simulink model "ChristmasLights"  (R2021a)
settings: Solver=FixedStepDiscrete  StartTime=0.0  StopTime=40.0  FixedStep=0.050  RelTol=1e-3
settings Model: EnablePacing=on  Creator=ncleju  LastModifiedBy=ncleju

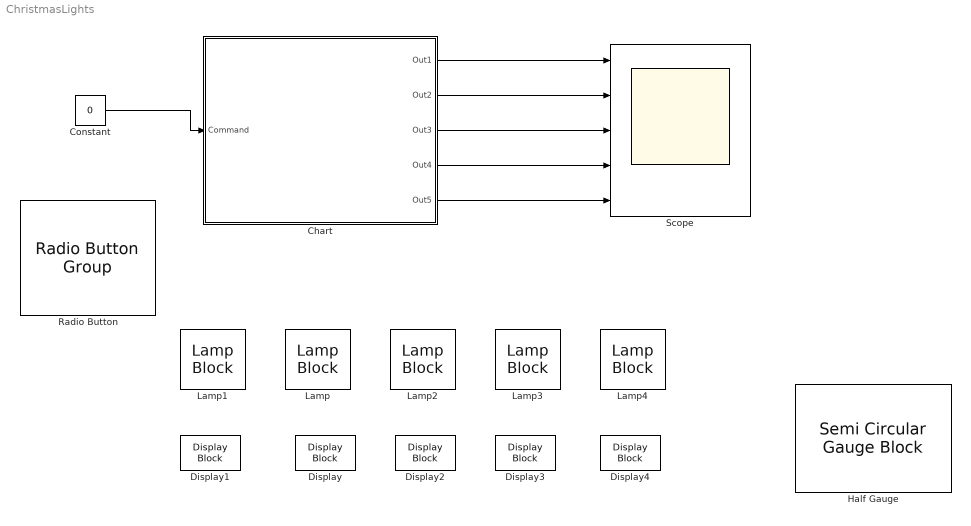
== system ChristmasLights ==
  Chart : Stateflow chart  TreatAsAtomicUnit=on
  Constant : Constant  Value=0
  Display{,1..4} (5 alike) : DisplayBlock  LabelPosition=Hide  Format=short  Transparency=1
  Half Gauge : SemiCircularGaugeBlock
  Lamp{,1..4} (5 alike) : LampBlock
  Radio Button : RadioButtonGroup  SelectedLabel=Cyclic  ButtonGroupName=Group
      settings: Values={{'Flash', 'Slow', 'Train', 'Cyclic'}, [1 2 3 0]}
  Scope : Scope  NumInputPorts=5
  wires:
  Chart/3(Out3) -> Scope/3
  Chart/4(Out4) -> Scope/4
  Chart/5(Out5) -> Scope/5
  Constant/1 -> Chart/1(Command)
  Chart/1(Out1) -> Scope/1
  Chart/2(Out2) -> Scope/2

== stateflow chart ChristmasLights/Chart ==
  state WORKING
    (history)
    state SLOW
      state INCREASE
      state DECREASE
        du:
        Out1 = Out1 - 1.66;
        Out2 = Out2 - 1.66;
        Out3 = Out3 - 1.66;
        Out4 = Out4 - 1.66;
        Out5 = Out5 - 1.66;
      (default) -> INCREASE : {Out1 = 0;
          | Out2 = 0;
          | Out3 = 0;
          | Out4 = 0;
          | Out5 = 0;}
      INCREASE -> DECREASE [order 1] : [Out1 >= 100]
      INCREASE -> INCREASE [order 2] : {Out1 = Out1 + 1.66;
          | Out2 = Out2 + 1.66;
          | Out3 = Out3 + 1.66;
          | Out4 = Out4 + 1.66;
          | Out5 = Out5 + 1.66;}
      DECREASE -> INCREASE : [Out1<=0]
    state FLASH
      state OFF
        en:
        Out1 = 0;
        Out2 = 0;
        Out3 = 0;
        Out4 = 0;
        Out5 = 0;
      state ON
        en:
        Out1 = 100;
        Out2 = 100;
        Out3 = 100;
        Out4 = 100;
        Out5 = 100;
      (default) -> OFF
      OFF -> ON : [after(0.2, sec)]
      ON -> OFF : [after(0.2, sec)]
    state TRAIN
      state L1
        en:
        Out1 = 100;
        Out2 = 0;
        Out3 = 0;
        Out4 = 0;
        Out5 = 0;
      state L2
        en:
        Out1 = 0;
        Out2 = 100;
        Out3 = 0;
        Out4 = 0;
        Out5 = 0;
      state L3
        en:
        Out1 = 0;
        Out2 = 0;
        Out3 = 100;
        Out4 = 0;
        Out5 = 0;
      state L4
        en:
        Out1 = 0;
        Out2 = 0;
        Out3 = 0;
        Out4 = 100;
        Out5 = 0;
      state L5
        en:
        Out1 = 0;
        Out2 = 0;
        Out3 = 0;
        Out4 = 0;
        Out5 = 100;
      (default) -> L1
      L4 -> L5 : [after(250,msec)]
      L5 -> (junction 50)
      L3 -> L4 : [after(250,msec)]
      L2 -> L3 : [after(250,msec)]
      L1 -> L2 : [after(250,msec)]
      (junction 51) -> L1
      (junction 50) -> (junction 51) : [after(250,msec)]
    (default) -> (junction 24)
    (junction 24) -> SLOW [order 2] : [Command == 2]
    (junction 24) -> FLASH [order 1] : [Command == 1]
    (junction 24) -> FLASH [order 4]
    (junction 24) -> TRAIN [order 3] : [Command == 3]
    FLASH -> SLOW [order 1] : [Command == 2]
    SLOW -> FLASH [order 1] : [Command == 1]
    FLASH -> SLOW [order 2] : [after(10, sec) && Command == 0]
    TRAIN -> FLASH [order 1] : [Command == 1]
    FLASH -> TRAIN [order 3] : [Command == 3]
    TRAIN -> FLASH [order 3] : [after(10, sec) && Command == 0]
    SLOW -> TRAIN [order 3] : [after(10, sec) && Command == 0]
    TRAIN -> SLOW [order 2] : [Command == 2]
    SLOW -> TRAIN [order 2] : [Command == 3]
  state PAUSE
    en:
    Out1 = 0;
    Out2 = 0;
    Out3 = 0;
    Out4 = 0;
    Out5 = 0;
  (default) -> WORKING
  WORKING -> PAUSE : [Overheating == true]
  PAUSE -> WORKING : [Overheating == false && after(15, sec)]
  data: Out1 output; Out2 output; Out3 output; Out4 output; Out5 output; Command input
